simulink model "Simulation_WTA"  (R2020a)
settings: Solver=ode45  StartTime=0.0  StopTime=100  RelTol=1e-3  EnableMultiTasking=on
undefined symbols (not defined in the file): n
(part 1 of 5)
settings Model: Creator=LVQ  LastModifiedBy=levie
settings DataIOCC: LimitDataPoints=on  SaveFormat=Array  ReturnWorkspaceOutputs=off
settings OptimizationCC: LifeSpan=inf
settings DebuggingCC: SolverPrmCheckMsg=warning  SFUnexpectedBacktrackingDiag=warning  SFNoUnconditionalDefaultTransitionDiag=warning  SFExecutionAtInitializationDiag=none  ArithmeticOperatorsInVariantConditions=warning
settings HardwareCC: ProdBitPerPointer=32  ProdBitPerSizeT=32  ProdBitPerPtrDiffT=32  ProdLargestAtomicFloat=None  ProdIntDivRoundTo=Undefined  ProdEndianess=Unspecified  ProdWordSize=32  ProdHWDeviceType=32-bit Generic
settings ModelReferenceCC: PropagateSignalLabelsOutOfModel=off
settings SFSimCC: SimUseLocalCustomCode=off  CustomCodeUndefinedFunction=UseInterfaceOnly
settings RTWCC: RTWUseLocalCustomCode=off
settings CodeAppCC: StateflowObjectComments=on
settings GRTTargetCC: TargetLangStandard=C89/C90 (ANSI)
settings ConfigComp: CovMetricSettings=dw  CovHtmlReporting=on  CovSaveCumulativeToWorkspaceVar=on  CovSaveSingleToWorkspaceVar=on  CovExternalEMLEnable=off  CovSFcnEnable=off

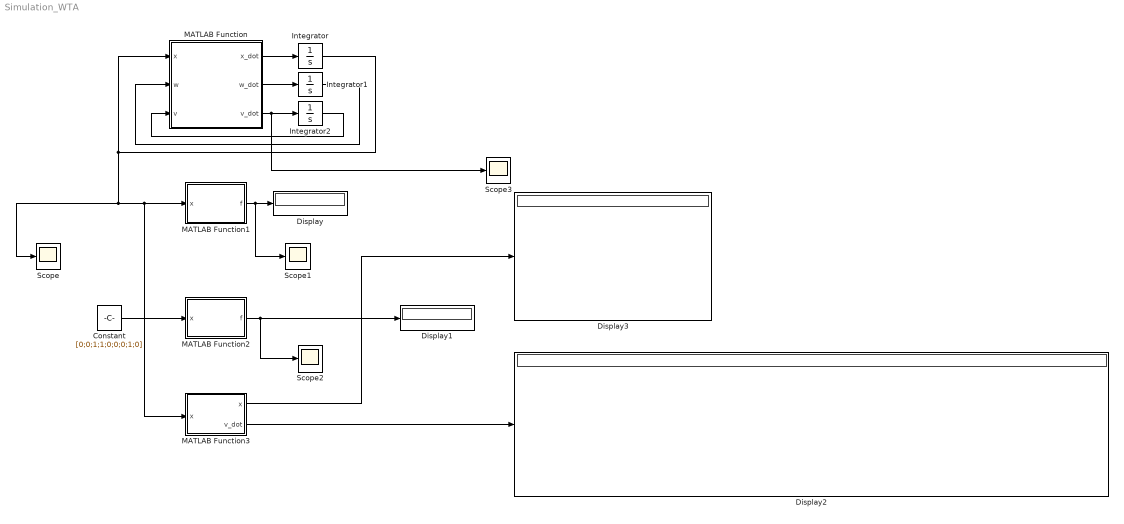
== system Simulation_WTA ==
  Constant : Constant  Value=[0;0;1;1;0;0;0;1;0]
  Display{,1..3} (4 alike) : Display
  Integrator : Integrator  InitialCondition=zeros(n*n,1)
  Integrator1 : Integrator  InitialCondition=ones(n*n,1)
  Integrator2 : Integrator  InitialCondition=ones(2*n,1)
  MATLAB Function : MATLAB Function  TreatAsAtomicUnit=on
  MATLAB Function1 : MATLAB Function  TreatAsAtomicUnit=on
  MATLAB Function2 : MATLAB Function  TreatAsAtomicUnit=on
  MATLAB Function3 : MATLAB Function  TreatAsAtomicUnit=on
  Scope{,1..3} (4 alike) : Scope
  wires:
  MATLAB Function/1(x_dot) -> Integrator/1
  MATLAB Function/2(w_dot) -> Integrator1/1
  MATLAB Function/3(v_dot) -> Scope3/1, Integrator2/1
  Integrator/1 -> Scope/1, MATLAB Function3/1("x "), MATLAB Function1/1(x), MATLAB Function/1(x)
  Integrator1/1 -> MATLAB Function/2(w)
  Integrator2/1 -> MATLAB Function/3(v)
  MATLAB Function1/1(f) -> Scope1/1, Display/1
  MATLAB Function2/1(f) -> Scope2/1, Display1/1
  MATLAB Function3/2(v_dot) -> Display2/1
  MATLAB Function3/1(x) -> Display3/1
  Constant/1 -> MATLAB Function2/1(x)
